simulink model "sampleModel1413"  (R2023a)
settings: Solver=VariableStepAuto  StartTime=0.0  StopTime=10.0  RelTol=1e-3
libraries: hdlsllib x4, simulink x3
settings Model: Creator=user1  LastModifiedBy=user1

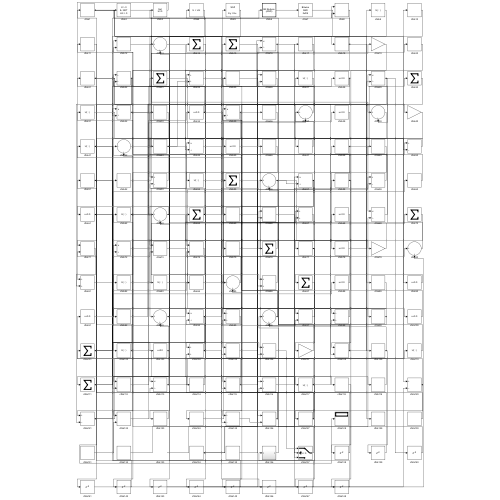
[thumbnail: Simulink's stored preview of the top-level diagram]
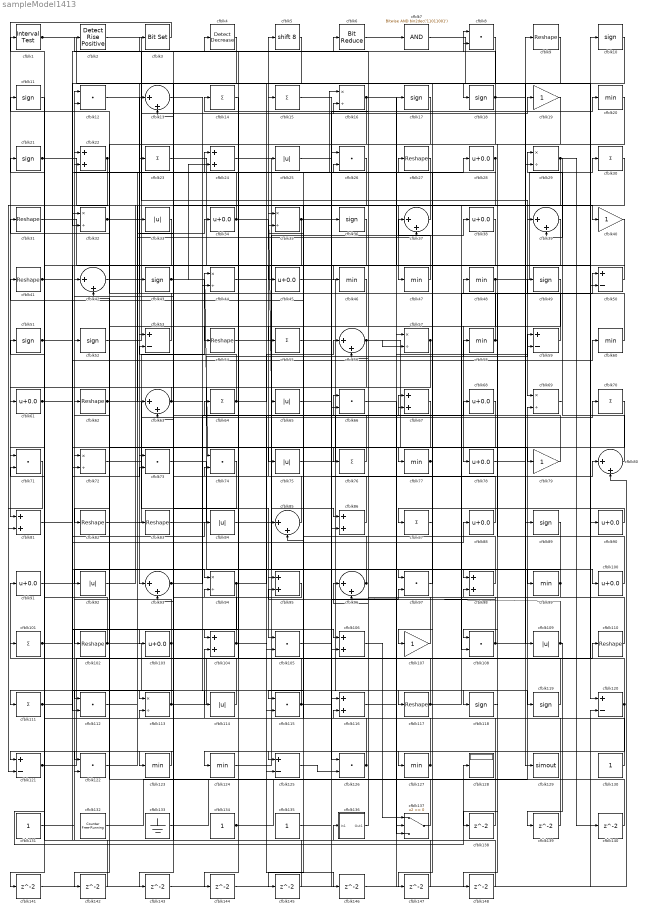
== system sampleModel1413 ==
  cfblk1 : hdlsllib/Logic and Bit Operations/Interval Test  IntervalClosedRight=on  uplimit=0.5  IntervalClosedLeft=on  lowlimit=-0.5  OutDataTypeStr=boolean
  cfblk{10..11,17..18,21,36,43,49,51..52,89,118..119} (13 alike) : Signum
  cfblk{28,34,38,45,61,68,78,88,90..91,100,103} (12 alike) : Bias  Bias=0.0  SaturateOnIntegerOverflow=off
  cfblk{14..15,23,30,55,64,70,76,87,101,111} (11 alike) : Sum  Inputs=+
  cfblk{9,27,31,41,54,62,82..83,102,110,117} (11 alike) : Reshape
  cfblk{22,24,67,81,86,95,98,104,106,116} (10 alike) : Sum
  cfblk{8,12,26,66,71,73..74,97,105,108,112,115,122,126} (14 alike) : DotProduct  OutDataTypeStr=Inherit: Inherit via internal rule
  cfblk{19,40,79,107} (4 alike) : Gain
  cfblk{25,33,65,75,84,92,109,114} (8 alike) : Abs  SaturateOnIntegerOverflow=off
  cfblk{16,29,32,35,44,57,69,72,94,113} (10 alike) : Product  Inputs=*/  RndMeth=Zero  SaturateOnIntegerOverflow=on
  cfblk{50,53,59,120..121,125} (6 alike) : Sum  Inputs=+-
  cfblk{20,46..48,58,60,77,99,123..124,127} (11 alike) : MinMax
  cfblk128 : Display
  cfblk129 : ToWorkspace  VariableName=simout  SaveFormat=Timeseries  SampleTime=-1
  cfblk{13,37,39,42,56,63,80,85,93,96} (10 alike) : Sum  Inputs=|++
  cfblk{130..131,134..135} (4 alike) : Constant  SampleTime=-1
  cfblk132 : hdlsllib/Sources/Counter Free-Running  NumBits=16  tsamp=-1
  cfblk133 : Ground
  cfblk136 : Subsystem
      settings: LibrarySourceBlock=|
      | hdlsllib/Ports &
      | Subsystems/Subsystem
  cfblk137 : Switch  SaturateOnIntegerOverflow=off  InputSameDT=off
  cfblk{138..148} (11 alike) : Delay  SampleTime=1
  cfblk2 : hdlsllib/Logic and Bit Operations/Detect Rise Positive  vinit=0  OutDataTypeStr=boolean
  cfblk3 : simulink/Logic and Bit Operations/Bit Set  iBit=0
      settings: LibrarySourceBlock=|
      | hdlsllib/Logic and Bit
      | Operations/Bit Set
  cfblk4 : simulink/Logic and Bit Operations/Detect Decrease  vinit=0.0  OutDataTypeStr=boolean
      settings: LibrarySourceBlock=|
      | hdlsllib/Logic and Bit
      | Operations/Detect
      | Decrease
  cfblk5 : ArithShift  BitShiftNumber=8
  cfblk6 : hdlsllib/Logic and Bit Operations/Bit Reduce  mode=AND
  cfblk7 : simulink/Logic and Bit Operations/Bitwise Operator  logicop=AND  UseBitMask=on  BitMask=bin2dec('11011001')  BitMaskRealWorld=Stored Integer
      settings: LibrarySourceBlock=|
      | hdlsllib/Logic and Bit
      | Operations/Bitwise
      | Operator
  wires:
  cfblk103/1 -> cfblk12/1, cfblk122/1
  cfblk35/1 -> cfblk93/1, cfblk39/1
  cfblk28/1 -> cfblk22/2, cfblk144/1
  cfblk106/1 -> cfblk137/1
  cfblk92/1 -> cfblk47/1
  cfblk2/1 -> cfblk69/1
  cfblk131/1 -> cfblk52/1
  cfblk6/1 -> cfblk7/1
  cfblk117/1 -> cfblk136/1(In1), cfblk74/2, cfblk50/1
  cfblk3/1 -> cfblk81/1
  cfblk79/1 -> cfblk42/1
  cfblk11/1 -> cfblk128/1
  cfblk133/1 -> cfblk69/2
  cfblk82/1 -> cfblk70/1
  cfblk49/1 -> cfblk78/1
  cfblk88/1 -> cfblk5/1
  cfblk60/1 -> cfblk31/1
  cfblk27/1 -> cfblk16/1
  cfblk42/1 -> cfblk19/1
  cfblk124/1 -> cfblk38/1
  cfblk52/1 -> cfblk6/1
  cfblk75/1 -> cfblk68/1
  cfblk48/1 -> cfblk30/1, cfblk145/1
  cfblk12/1 -> cfblk18/1
  cfblk73/1 -> cfblk100/1
  cfblk37/1 -> cfblk15/1
  cfblk5/1 -> cfblk123/1
  cfblk91/1 -> cfblk72/1
  cfblk15/1 -> cfblk126/1
  cfblk83/1 -> cfblk59/1
  cfblk17/1 -> cfblk102/1
  cfblk127/1 -> cfblk62/1, cfblk104/2
  cfblk45/1 -> cfblk117/1
  cfblk57/1 -> cfblk83/1, cfblk104/1
  cfblk31/1 -> cfblk90/1
  cfblk59/1 -> cfblk11/1
  cfblk89/1 -> cfblk113/1
  cfblk54/1 -> cfblk98/1
  cfblk110/1 -> cfblk14/1
  cfblk90/1 -> cfblk87/1
  cfblk69/1 -> cfblk49/1
  cfblk87/1 -> cfblk127/1
  cfblk102/1 -> cfblk137/2, cfblk21/1
  cfblk86/1 -> cfblk4/1
  cfblk101/1 -> cfblk26/2, cfblk88/1, cfblk84/1
  cfblk4/1 -> cfblk53/1
  cfblk47/1 -> cfblk37/1
  cfblk121/1 -> cfblk110/1, cfblk73/2
  cfblk99/1 -> cfblk98/2, cfblk92/1
  cfblk62/1 -> cfblk105/1, cfblk34/1
  cfblk24/1 -> cfblk99/1
  cfblk97/1 -> cfblk27/1
  cfblk41/1 -> cfblk103/1, cfblk114/1
  cfblk1/1 -> cfblk120/1, cfblk115/2, cfblk125/2
  cfblk34/1 -> cfblk65/1, cfblk12/2
  cfblk16/1 -> cfblk82/1, cfblk50/2
  cfblk98/1 -> cfblk35/1
  cfblk84/1 -> cfblk86/1
  cfblk107/1 -> cfblk66/1
  cfblk125/1 -> cfblk126/2
  cfblk38/1 -> cfblk93/2
  cfblk112/1 -> cfblk37/2
  cfblk72/1 -> cfblk44/1
  cfblk122/1 -> cfblk28/1
  cfblk53/1 -> cfblk13/1
  cfblk21/1 -> cfblk63/1, cfblk108/2
  cfblk114/1 -> cfblk91/1
  cfblk43/1 -> cfblk74/1, cfblk24/2
  cfblk71/1 -> cfblk81/2
  cfblk123/1 -> cfblk121/1
  cfblk81/1 -> cfblk106/1
  cfblk32/1 -> cfblk16/2, cfblk40/1
  cfblk115/1 -> cfblk24/1, cfblk20/1
  cfblk10/1 -> cfblk77/1
  cfblk25/1 -> cfblk79/1
  cfblk126/1 -> cfblk53/2, cfblk71/2
  cfblk76/1 -> cfblk64/1
  cfblk8/1 -> cfblk32/2
  cfblk23/1 -> cfblk45/1
  cfblk68/1 -> cfblk112/1
  cfblk108/1 -> cfblk9/1, cfblk2/1, cfblk95/2
  cfblk65/1 -> cfblk58/1
  cfblk61/1 -> cfblk106/2, cfblk76/1
  cfblk94/1 -> cfblk112/2, cfblk67/1
  cfblk116/1 -> cfblk59/2
  cfblk77/1 -> cfblk97/1, cfblk147/1
  cfblk113/1 -> cfblk111/1, cfblk10/1
  cfblk105/1 -> cfblk80/1
  cfblk119/1 -> cfblk25/1
  cfblk55/1 -> cfblk116/1
  cfblk18/1 -> cfblk129/1, cfblk86/2, cfblk8/1
  cfblk51/1 -> cfblk94/1, cfblk118/1
  cfblk13/1 -> cfblk119/1
  cfblk120/1 -> cfblk101/1, cfblk124/1
  cfblk70/1 -> cfblk107/1
  cfblk36/1 -> cfblk72/2
  cfblk64/1 -> cfblk56/1, cfblk23/1
  cfblk100/1 -> cfblk48/1
  cfblk66/1 -> cfblk137/3
  cfblk67/1 -> cfblk105/2
  cfblk132/1 -> cfblk36/1
  cfblk44/1 -> cfblk85/1
  cfblk95/1 -> cfblk94/2
  cfblk136/1(Out1) -> cfblk116/2
  cfblk9/1 -> cfblk73/1
  cfblk7/1 -> cfblk89/1
  cfblk29/1 -> cfblk55/1, cfblk39/2, cfblk140/1
  cfblk50/1 -> cfblk46/1
  cfblk33/1 -> cfblk43/1
  cfblk80/1 -> cfblk29/1
  cfblk104/1 -> cfblk22/1, cfblk146/1
  cfblk134/1 -> cfblk17/1, cfblk66/2
  cfblk63/1 -> cfblk75/1, cfblk61/1
  cfblk109/1 -> cfblk96/2, cfblk139/1
  cfblk93/1 -> cfblk3/1, cfblk67/2
  cfblk30/1 -> cfblk125/1
  cfblk20/1 -> cfblk44/2
  cfblk137/1 -> cfblk42/2
  cfblk40/1 -> cfblk115/1
  cfblk58/1 -> cfblk13/2, cfblk108/1
  cfblk130/1 -> cfblk85/2
  cfblk85/1 -> cfblk33/1
  cfblk22/1 -> cfblk121/2, cfblk71/1
  cfblk56/1 -> cfblk109/1, cfblk95/1, cfblk57/2
  cfblk111/1 -> cfblk60/1, cfblk8/2
  cfblk14/1 -> cfblk54/1
  cfblk135/1 -> cfblk97/2
  cfblk96/1 -> cfblk35/2, cfblk41/1
  cfblk78/1 -> cfblk29/2
  cfblk26/1 -> cfblk63/2
  cfblk19/1 -> cfblk138/1
  cfblk138/1 -> cfblk1/1
  cfblk139/1 -> cfblk56/2
  cfblk140/1 -> cfblk96/1
  cfblk39/1 -> cfblk141/1
  cfblk141/1 -> cfblk80/2
  cfblk46/1 -> cfblk142/1
  cfblk142/1 -> cfblk32/1
  cfblk74/1 -> cfblk143/1
  cfblk143/1 -> cfblk120/2
  cfblk144/1 -> cfblk26/1
  cfblk145/1 -> cfblk122/2
  cfblk146/1 -> cfblk57/1
  cfblk147/1 -> cfblk113/2
  cfblk118/1 -> cfblk148/1
  cfblk148/1 -> cfblk51/1

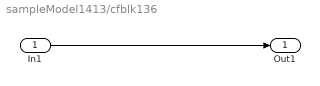
== system sampleModel1413/cfblk136 ==
  In1 : Inport
  Out1 : Outport
  wires:
  In1/1 -> Out1/1
